simulink model "Sub2_2023"  (R2023b)
settings: Solver=FixedStepDiscrete  StartTime=0.0  StopTime=4.5  FixedStep=7.5e-05  RelTol=1e-3  EnableMultiTasking=on
undefined symbols (not defined in the file or in its folder): D1, D11, Delta
libraries: spsSeriesRLCBranchLib x41, spsLoadFlowBusLib x29, spsDistributedParametersLineLib x19, spsThreePhaseSeriesRLCLoadLib x15, spsThreePhaseTransformerTwoWindingsLib x13, spsThreePhaseParallelRLCLoadLib x11, spsThreePhaseVIMeasurementLib x11, spsSynchronousMachinepuStandardLib x7, spsExcitationSystemLib x7, spsHydraulicTurbineandGovernorLib x7, spsGenericPowerSystemStabilizerLib x7, spsMultiBandPowerSystemStabilizerLib x7
(part 2 of 5)

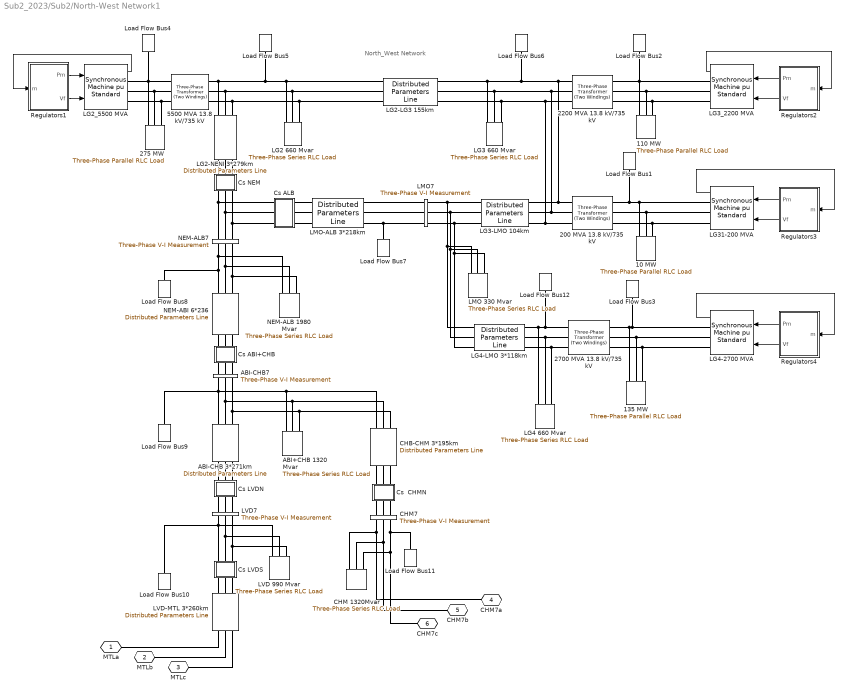
== system Sub2_2023/Sub2/North-West Network1 ==
  note: North_West Network
  10 MW : spsThreePhaseParallelRLCLoadLib/Three-Phase Parallel RLC Load  LConnTagsString=A|B|C  Configuration=Y (grounded)  NominalVoltage=(13800)*1  Vabc=[1e3 1e3 1e3]  Vabcp=[1e3 1e3 1e3]  NominalFrequency=60  UnbalancedPower=off  ActivePower=10000000  InductivePower=0  CapacitivePower=0  Pabc=[10e3 9e3 11e3]  QLabc=[100 90 110]  QCabc=[100 90 110]  Pabcp=[10e3 9e3 11e3]  QLabcp=[100 90 110]  QCabcp=[100 90 110]  Measurements=None  LoadType=constant PQ
  110 MW : spsThreePhaseParallelRLCLoadLib/Three-Phase Parallel RLC Load  LConnTagsString=A|B|C  Configuration=Y (grounded)  NominalVoltage=(13800)*1  Vabc=[1e3 1e3 1e3]  Vabcp=[1e3 1e3 1e3]  NominalFrequency=60  UnbalancedPower=off  ActivePower=110000000  InductivePower=0  CapacitivePower=0  Pabc=[10e3 9e3 11e3]  QLabc=[100 90 110]  QCabc=[100 90 110]  Pabcp=[10e3 9e3 11e3]  QLabcp=[100 90 110]  QCabcp=[100 90 110]  Measurements=None  LoadType=constant PQ
  135 MW : spsThreePhaseParallelRLCLoadLib/Three-Phase Parallel RLC Load  LConnTagsString=A|B|C  Configuration=Y (grounded)  NominalVoltage=(13800)*1  Vabc=[1e3 1e3 1e3]  Vabcp=[1e3 1e3 1e3]  NominalFrequency=60  UnbalancedPower=off  ActivePower=135000000  InductivePower=0  CapacitivePower=0  Pabc=[10e3 9e3 11e3]  QLabc=[100 90 110]  QCabc=[100 90 110]  Pabcp=[10e3 9e3 11e3]  QLabcp=[100 90 110]  QCabcp=[100 90 110]  Measurements=None  LoadType=constant PQ
  200 MVA 13.8 kV/735 kV : spsThreePhaseTransformerTwoWindingsLib/Three-Phase Transformer (Two Windings)  Winding1Connection=Delta (D1)  Winding2Connection=Yg  CoreType=Three single-phase transformers  SetSaturation=off  Hysteresis=off  DataFile='basic_model'  SetInitialFlux=off  Measurements=None  UNITS=pu  NominalPower=[ 200e6 60 ]  Winding1="[ 13.8e3 0.002  0.0]"  Winding2=[ 735e3 0.002 0.12]  Rm=500  Lm=500  L0=0.5  Saturation="[ 0,0  ;  0.005,1.2  ;  1.0,1.4 ]"  InitialFluxes=[ 0.8 , -0.8 , 0.7 ]  BreakLoop=off  DiscreteSolver=Trapezoidal iterative  DataType=off  TransfoNumber=0
  2200 MVA 13.8 kV/735 kV : spsThreePhaseTransformerTwoWindingsLib/Three-Phase Transformer (Two Windings)  Winding1Connection=Delta (D1)  Winding2Connection=Yg  CoreType=Three single-phase transformers  SetSaturation=off  Hysteresis=off  DataFile='basic_model'  SetInitialFlux=off  Measurements=None  UNITS=pu  NominalPower=[ 2200e6 60 ]  Winding1="[ 13.8e3 0.002  0.0]"  Winding2=[ 735e3 0.002 0.12]  Rm=500  Lm=500  L0=0.5  Saturation="[ 0,0  ;  0.005,1.2  ;  1.0,1.4 ]"  InitialFluxes=[ 0.8 , -0.8 , 0.7 ]  BreakLoop=off  DiscreteSolver=Trapezoidal iterative  DataType=off  TransfoNumber=0
  2700 MVA 13.8 kV/735 kV : spsThreePhaseTransformerTwoWindingsLib/Three-Phase Transformer (Two Windings)  Winding1Connection=Delta (D1)  Winding2Connection=Yg  CoreType=Three single-phase transformers  SetSaturation=off  Hysteresis=off  DataFile='basic_model'  SetInitialFlux=off  Measurements=None  UNITS=pu  NominalPower=[ 2700e6 60 ]  Winding1="[ 13.8e3 0.002  0.0]"  Winding2=[ 735e3 0.002 0.12]  Rm=500  Lm=500  L0=0.5  Saturation="[ 0,0  ;  0.005,1.2  ;  1.0,1.4 ]"  InitialFluxes=[ 0.8 , -0.8 , 0.7 ]  BreakLoop=off  DiscreteSolver=Trapezoidal iterative  DataType=off  TransfoNumber=0
  275 MW : spsThreePhaseParallelRLCLoadLib/Three-Phase Parallel RLC Load  LConnTagsString=A|B|C  Configuration=Y (grounded)  NominalVoltage=(13800)*1  Vabc=[1e3 1e3 1e3]  Vabcp=[1e3 1e3 1e3]  NominalFrequency=60  UnbalancedPower=off  ActivePower=275000000  InductivePower=0  CapacitivePower=0  Pabc=[10e3 9e3 11e3]  QLabc=[100 90 110]  QCabc=[100 90 110]  Pabcp=[10e3 9e3 11e3]  QLabcp=[100 90 110]  QCabcp=[100 90 110]  Measurements=None  LoadType=constant PQ
  5500 MVA 13.8 kV/735 kV : spsThreePhaseTransformerTwoWindingsLib/Three-Phase Transformer (Two Windings)  Winding1Connection=Delta (D1)  Winding2Connection=Yg  CoreType=Three single-phase transformers  SetSaturation=off  Hysteresis=off  DataFile='basic_model'  SetInitialFlux=off  Measurements=None  UNITS=pu  NominalPower=[ 5500e6 60 ]  Winding1="[ 13.8e3 0.002  0.0]"  Winding2=[ 735e3 0.002 0.12]  Rm=500  Lm=500  L0=0.5  Saturation="[ 0,0  ;  0.005,1.2  ;  1.0,1.4 ]"  InitialFluxes=[ 0.8 , -0.8 , 0.7 ]  BreakLoop=off  DiscreteSolver=Trapezoidal iterative  DataType=off  TransfoNumber=0
  ABI+CHB 1320 Mvar : spsThreePhaseSeriesRLCLoadLib/Three-Phase Series RLC Load  LConnTagsString=A|B|C  Configuration=Y (grounded)  NominalVoltage=735e3  Vabc=[1e3 1e3 1e3]  Vabcp=[1e3 1e3 1e3]  NominalFrequency=60  UnbalancedPower=off  ActivePower=4400000  InductivePower=1320e6  CapacitivePower=0  Pabc=[10e3 9e3 11e3]  QLabc=[100 90 110]  QCabc=[100 90 110]  Pabcp=[10e3 9e3 11e3]  QLabcp=[100 90 110]  QCabcp=[100 90 110]  Measurements=None  LoadType=constant Z
  ABI-CHB 3*271km : spsDistributedParametersLineLib/Distributed Parameters Line  Phases=3  Length=271  Frequency=60  Resistance="[0.01273  0.3864]/3"  Inductance="[0.9337e-3  4.1264e-3]/3"  Capacitance=[12.74e-9 7.751e-9]*3  x1=[-0.001575 2.6660325112539e-08 -34814.2579740654 -747194.944178159;-0.0015 2.67772386504407e-08 -13676.7298713687 -747880.497252828;-0.001425 2.68727468734707e-08 7471.73119992629 -747968.206100949;-0.00135 2.69467734338169e-08 28614.2194836213 -747458.00060941;-0.001275 2.69992591557795e-08 49733.8339980734 -746350.288628675;-0.0012 2.70301620830755e-08 70813.6920465805 -744645.955646752;-0.001125 2.70394575123777e-08 91836.9427131515 -742346.36408135;-0.00105 2.7027138013062e-08 112786.78033287 -739453.352190782;-0.000975 2.69932134331478e-08 133646.457926086 -735969.232604489;-0.0009 2.69377108914251e-08 154399.300585695 -731896.790474358;-0.000825 2.68606747557766e-08 175028.718806805 -727239.281248318;-0.00075 2.67621666077105e-08 195518.221748129 -722000.428067983;-0.000675 2.6642265193133e-08 215851.430414517 -716184.418792427;-0.0006 2.65010663594005e-08 236012.09075007 -709795.902650478;-0.000525 2.63386829787002e-08 255984.086631383 -702839.986524191;-0.00045 2.6155244857822e-08 275751.45275053 -695322.230866489;-0.000375 2.59508986343932e-08 295298.387377488 -687248.64525622;-0.0003 2.57258076596581e-08 314609.264991793 -678625.683594189;-0.000225 2.5480151867898e-08 333668.648773346 -669460.238944015;-0.00015 2.5214127632594e-08 352461.302942372 -659759.638021913;-7.5e-05 2.49279476094497e-08 370972.204938665 -649531.635339838]  x2=[-0.001575 6.10028275120772e-08 -284619.341076116 -691578.75825678;-0.0015 6.12059670998859e-08 -264954.25531131 -699348.683851085;-0.001425 6.13601795740777e-08 -245077.369168744 -706559.560807914;-0.00135 6.14653416595602e-08 -225004.571927074 -713205.624862556;-0.001275 6.15213692913713e-08 -204751.909473291 -719281.563253095;-0.0012 6.15282176818794e-08 -184335.571475885 -724782.518967347;-0.001125 6.1485881356586e-08 -163771.878443069 -729704.09462548;-0.00105 6.13943941585016e-08 -143077.268676419 -734042.355995217;-0.000975 6.12538292210926e-08 -122268.285130346 -737793.835136796;-0.0009 6.10642989098193e-08 -101361.562187906 -740955.533175191;-0.000825 6.08259547323125e-08 -80373.8123635378 -743524.922697366;-0.00075 6.05389872172611e-08 -59321.8129433265 -745499.949772649;-0.000675 6.02036257621058e-08 -38222.3925735024 -746879.035594615;-0.0006 5.98201384496626e-08 -17092.4178078773 -747661.077743159;-0.000525 5.93888318338216e-08 4051.22037502064 -747845.451065755;-0.00045 5.89100506944922e-08 25191.6200743366 -747432.008177186;-0.000375 5.83841777619916e-08 46311.8819780098 -746421.079577375;-0.0003 5.7811633411096e-08 67395.1228718253 -744813.473387174;-0.000225 5.71928753249992e-08 88424.4891355971 -742610.474702377;-0.00015 5.65283981294479e-08 109383.170215694 -739813.844566423;-7.5e-05 5.58187329973454e-08 130254.412063139 -736425.818562655]  x3=[-0.001575 1.20876651145068e-10 -354.964030660806 -109.750554356937;-0.0015 1.28668645904503e-10 -351.719210477191 -119.74113184108;-0.001425 1.36357784917099e-10 -348.193231338204 -129.635990096531;-0.00135 1.43937921602775e-10 -344.388911857622 -139.427219324996;-0.001275 1.51402996516247e-10 -340.309293150227 -149.106992567641;-0.0012 1.58747042190847e-10 -335.957636400794 -158.66757196184;-0.001125 1.65964187908831e-10 -331.337420257147 -168.101314926709;-0.00105 1.73048664394338e-10 -326.452338049379 -177.400680272461;-0.000975 1.79994808425261e-10 -321.306294837463 -186.558234228725;-0.0009 1.86797067360342e-10 -315.903404289605 -195.566656386983;-0.000825 1.93450003577867e-10 -310.247985393842 -204.418745552396;-0.00075 1.99948298822415e-10 -304.344559005508 -213.107425500326;-0.000675 2.06286758456196e-10 -298.197844233333 -221.625750632964;-0.0006 2.12460315611561e-10 -291.812754667058 -229.966911531533;-0.000525 2.18464035241378e-10 -285.194394449587 -238.124240399636;-0.00045 2.24293118064034e-10 -278.348054196814 -246.091216393387;-0.000375 2.2994290439991e-10 -271.279206768384 -253.861470834074;-0.0003 2.35408877896253e-10 -263.993502892774 -261.428792299187;-0.000225 2.40686669137482e-10 -256.496766650188 -268.787131587732;-0.00015 2.45772059138033e-10 -248.794990816874 -275.930606555866;-7.5e-05 2.50660982714947e-10 -240.894332074591 -282.853506818999]  x4=[-0.001575 1.8611765414938e-10 -5971.27343085196 -15054.8004559038;-0.0015 1.8231186212515e-10 -5543.27939856525 -15217.5948036283;-0.001425 1.78360332787803e-10 -5110.85415354235 -15368.2244389038;-0.00135 1.7426622492943e-10 -4674.3433699078 -15506.5689507045;-0.001275 1.70032811317211e-10 -4234.0959877032 -15632.5177485445;-0.0012 1.65663476077214e-10 -3790.46393394987 -15745.9701508819;-0.001125 1.61161711989177e-10 -3343.80184132378 -15846.8354656021;-0.00105 1.56531117694433e-10 -2894.46676466762 -15935.0330625157;-0.000975 1.51775394819211e-10 -2442.81789556661 -16010.4924378134;-0.0009 1.46898345015611e-10 -1989.21627521625 -16073.1532704251;-0.000825 1.41903866922626e-10 -1534.02450581152 -16122.9654702398;-0.00075 1.36795953049626e-10 -1077.6064606882 -16159.8892181473;-0.000675 1.31578686584805e-10 -620.326993448138 -16183.8949978684;-0.0006 1.2625623813115e-10 -162.551646300836 -16194.9636195501;-0.000525 1.20832862372518e-10 295.353642145395 -16193.0862351056;-0.00045 1.1531289467251e-10 753.022829409158 -16178.2643452873;-0.000375 1.09700747608848e-10 1210.09006174473 -16150.5097984871;-0.0003 1.04000907446025e-10 1666.18996659994 -16109.844781265;-0.000225 9.82179305490565e-11 2120.95794468941 -16056.3018006137;-0.00015 9.2356439741192e-11 2574.03046144964 -15989.9236579727;-7.5e-05 8.64211206084993e-11 3025.04533764297 -15910.7634150135]  x5=0.00153261764655846  V1=ones(3,3)  V2=ones(3,3)  I1=ones(3,3)  I2=ones(3,3)  nHarmo=1  Measurements=None  Decoupling=on  VsMag0=[610743.955114517 610743.501375054 610743.958218176]  VrMag0=[610622.360478052 610622.247686738 610622.214003776]  VsAngle0=[1.35232982185072 -118.647645266053 121.352379141739]  VrAngle0=[-18.3496130787589 -138.349622838574 101.65039120684]  IsMag0=[305.299965910612 305.301188711725 305.286778309069]  IrMag0=[13308.3117169369 13308.3164139137 13308.324626215]  IsAngle0=[-68.7963830005534 171.200626740077 51.201923119545]  IrAngle0=[-17.6151010152162 -137.615048514482 102.384907722651]
      settings: AttributesFormatString=\n  LibrarySourceBlock=sps_lib/Power Grid Elements/Distributed Parameters Line
  ABI-CHB7 : spsThreePhaseVIMeasurementLib/Three-Phase V-I Measurement  VoltageMeasurement=no  SetLabelV=on  LabelV=Vabc_ABI7  Vpu=on  VpuLL=off  CurrentMeasurement=no  SetLabelI=off  LabelI=A1  Ipu=off  Pbase=100e6  Vbase=500e3  OutputType=Magnitude  PhasorSimulation=off  PSBequivalent=0
  CHB-CHM 3*195km : spsDistributedParametersLineLib/Distributed Parameters Line  Phases=3  Length=195  Frequency=60  Resistance="[0.01273  0.3864]/3"  Inductance="[0.9337e-3  4.1264e-3]/3"  Capacitance=[12.74e-9 7.751e-9]*3  x1=[-0.001125 2.70394575123777e-08 0 0;-0.00105 2.7027138013062e-08 0 0;-0.000975 2.69932134331478e-08 0 0;-0.0009 2.69377108914251e-08 0 0;-0.000825 2.68606747557766e-08 0 0;-0.00075 2.67621666077105e-08 0 0;-0.000675 2.6642265193133e-08 215851.430414517 -716184.418792427;-0.0006 2.65010663594005e-08 236012.09075007 -709795.902650478;-0.000525 2.63386829787002e-08 255984.086631383 -702839.986524191;-0.00045 2.6155244857822e-08 275751.45275053 -695322.230866489;-0.000375 2.59508986343932e-08 295298.387377488 -687248.64525622;-0.0003 2.57258076596581e-08 314609.264991793 -678625.683594189;-0.000225 2.5480151867898e-08 333668.648773346 -669460.238944015;-0.00015 2.5214127632594e-08 352461.302942372 -659759.638021913;-7.5e-05 2.49279476094497e-08 370972.204938665 -649531.635339838]  x2=[-0.001125 1.81955879149765e-08 0 0;-0.00105 1.81407188523757e-08 0 0;-0.000975 1.80713483766866e-08 0 0;-0.0009 1.79875319416061e-08 0 0;-0.000825 1.788933654871e-08 0 0;-0.00075 1.77768406938928e-08 0 0;-0.000675 1.76501343046197e-08 127559.107191254 -726636.134488586;-0.0006 1.75093186680396e-08 148050.539525875 -722739.535823254;-0.000525 1.73545063500179e-08 168423.622524448 -718265.19023127;-0.00045 1.71858211051527e-08 188662.070256143 -713216.674436042;-0.000375 1.7003397777848e-08 208749.704415501 -707598.024143851;-0.0003 1.68073821945204e-08 228670.467255128 -701413.730817772;-0.000225 1.65979310470281e-08 248408.434422006 -694668.738087267;-0.00015 1.63752117674137e-08 267947.827687183 -687368.437796323;-7.5e-05 1.61394023940615e-08 287273.027558647 -679518.665693294]  x3=[-0.001125 1.00783620494122e-10 0 0;-0.00105 9.8868424952397e-11 0 0;-0.000975 9.68741955045023e-11 0 0;-0.0009 9.48025263069462e-11 0 0;-0.000825 9.26550734203876e-11 0 0;-0.00075 9.04335534858069e-11 0 0;-0.000675 8.81397423522494e-11 771.180648774861 -4323.83757003592;-0.0006 8.57754736572388e-11 893.110598565651 -4300.3071890933;-0.000525 8.33426373609954e-11 1014.326609409 -4273.33920838062;-0.00045 8.08431782356307e-11 1134.7317830805 -4242.95518568905;-0.000375 7.82790943105266e-11 1254.22986952659 -4209.17940954143;-0.0003 7.56524352751409e-11 1372.72534380533 -4172.03887977642;-0.000225 7.29653008405173e-11 1490.12348244765 -4131.56328596526;-0.00015 7.02198390608084e-11 1606.33043917774 -4087.78498367834;-7.5e-05 6.74182446161539e-11 1721.25331993244 -4040.73896862067]  x4=[-0.001125 7.25791212501294e-11 0 0;-0.00105 7.52447889614668e-11 0 0;-0.000975 7.78503071397922e-11 0 0;-0.0009 8.03935929737397e-11 0 0;-0.000825 8.28726133995272e-11 0 0;-0.00075 8.52853867261566e-11 0 0;-0.000675 8.76299842195474e-11 979.606952616618 -12037.6056406833;-0.0006 8.99045316443367e-11 1319.52443201694 -12005.1005057423;-0.000525 9.2107210762115e-11 1658.38710377571 -11962.9986771411;-0.00045 9.42362607848977e-11 1995.9240862579 -11911.3338104375;-0.000375 9.62899797826721e-11 2331.86555756419 -11850.1472057353;-0.0003 9.82667260438942e-11 2665.94297122251 -11779.4877746702;-0.000225 1.00164919387848e-10 2997.88927085992 -11699.4120013102;-0.00015 1.01983042427818e-10 3327.43910368346 -11609.9838970034;-7.5e-05 1.03719641784064e-10 3654.32903259903 -11511.274949208]  x5=0.0011028060556417  V1=ones(3,3)  V2=ones(3,3)  I1=ones(3,3)  I2=ones(3,3)  nHarmo=1  Measurements=None  Decoupling=on  VsMag0=[610743.955114517 610743.501375054 610743.958218176]  VrMag0=[602368.350238914 602368.356498701 602368.322152315]  VsAngle0=[1.35232982185072 -118.647645266053 121.352379141739]  VrAngle0=[-5.46332293595899 -125.46332636454 114.536674834106]  IsMag0=[3602.61669203481 3602.60152789078 3602.59275066962]  IrMag0=[9906.44607872251 9906.45414351813 9906.46948058419]  IsAngle0=[-5.30716137482798 -125.307461802343 114.692897272079]  IrAngle0=[-10.7676510977574 -130.767521740253 109.23237318601]
      settings: AttributesFormatString=\n  LibrarySourceBlock=sps_lib/Power Grid Elements/Distributed Parameters Line
  CHM 1320Mvar : spsThreePhaseSeriesRLCLoadLib/Three-Phase Series RLC Load  LConnTagsString=A|B|C  Configuration=Y (grounded)  NominalVoltage=735e3  Vabc=[1e3 1e3 1e3]  Vabcp=[1e3 1e3 1e3]  NominalFrequency=60  UnbalancedPower=off  ActivePower=4400000  InductivePower=1320e6  CapacitivePower=0  Pabc=[10e3 9e3 11e3]  QLabc=[100 90 110]  QCabc=[100 90 110]  Pabcp=[10e3 9e3 11e3]  QLabcp=[100 90 110]  QCabcp=[100 90 110]  Measurements=None  LoadType=constant Z
  CHM7 : spsThreePhaseVIMeasurementLib/Three-Phase V-I Measurement  VoltageMeasurement=no  SetLabelV=on  LabelV=Vabc_CHM7  Vpu=on  VpuLL=off  CurrentMeasurement=no  SetLabelI=off  LabelI=A1  Ipu=off  Pbase=100e6  Vbase=735e3  OutputType=Magnitude  PhasorSimulation=off  PSBequivalent=0
  "Cs  CHMN " : Subsystem  mask{Xc=25/3}
      mask prompts: Xc "Condensator Reactance at  60Hz  (ohm):"
      mask help: Series Compensation
      mask init:
      | Cs=1/Xc/(2*pi*60);
      mask Display: disp('Cs')
  "Cs ABI+CHB " : Subsystem  mask{Xc=25/6}
      mask prompts: Xc "Condensator Reactance at  60Hz  (ohm):"
      mask help: Series Compensation
      mask init:
      | Cs=1/Xc/(2*pi*60);
      mask Display: disp('Cs')
  Cs ALB : Subsystem  mask{Xc=16/3}
      mask prompts: Xc "Reactance @ 60Hz du condensateur (ohm):"
      mask init:
      | Cs=1/Xc/(2*pi*60);
      mask Display: disp('Cs')
  "Cs LVDN " : Subsystem  mask{Xc=34/3}
      mask prompts: Xc "Condensator Reactance at  60Hz  (ohm):"
      mask help: Series Compensation
      mask init:
      | Cs=1/Xc/(2*pi*60);
      mask Display: disp('Cs')
  "Cs LVDS " : Subsystem  mask{Xc=34/3}
      mask prompts: Xc "Condensator Reactance at  60Hz  (ohm):"
      mask help: Series Compensation
      mask init:
      | Cs=1/Xc/(2*pi*60);
      mask Display: disp('Cs')
  "Cs NEM " : Subsystem  mask{Xc=16/3}
      mask prompts: Xc "Condensator Reactance at  60Hz  (ohm):"
      mask help: Series Compensation
      mask init:
      | Cs=1/Xc/(2*pi*60);
      mask Display: disp('Cs')
  LG2 660 Mvar : spsThreePhaseSeriesRLCLoadLib/Three-Phase Series RLC Load  LConnTagsString=A|B|C  Configuration=Y (grounded)  NominalVoltage=735e3  Vabc=[1e3 1e3 1e3]  Vabcp=[1e3 1e3 1e3]  NominalFrequency=60  UnbalancedPower=off  ActivePower=2200000  InductivePower=660e6  CapacitivePower=0  Pabc=[10e3 9e3 11e3]  QLabc=[100 90 110]  QCabc=[100 90 110]  Pabcp=[10e3 9e3 11e3]  QLabcp=[100 90 110]  QCabcp=[100 90 110]  Measurements=None  LoadType=constant Z
  LG2-LG3 155km : spsDistributedParametersLineLib/Distributed Parameters Line  Phases=3  Length=155  Frequency=60  Resistance="[0.01273  0.3864]"  Inductance="[0.9337e-3  4.1264e-3]"  Capacitance=[12.74e-9 7.751e-9]  x1=[-0.0009 4.79474772159392e-10 425726.576739838 -584301.004479771;-0.000825 5.22458298158404e-10 442074.911234261 -572031.872778104;-0.00075 5.65024178987748e-10 458069.857808617 -559305.46754972;-0.000675 6.0713838813357e-10 473698.630347344 -546131.962088236;-0.0006 6.48767260141446e-10 488948.735448804 -532521.887092359;-0.000525 6.89877517528037e-10 503807.982412312 -518486.122247798;-0.00045 7.30436297382596e-10 518264.492983201 -504035.887530215;-0.000375 7.70411177637078e-10 532306.710848112 -489182.734236149;-0.0003 8.09770202983843e-10 545923.410872936 -473938.535749081;-0.000225 8.48481910420242e-10 559103.708076017 -458315.478048038;-0.00015 8.8651535439966e-10 571837.066329435 -442326.049966306;-7.5e-05 9.2384013156891e-10 584113.30678143 -425983.033208046]  x2=[-0.0009 -3.11578283864764e-10 428602.512418884 -576982.581433748;-0.000825 -3.58188817976031e-10 444742.801992352 -564635.073574132;-0.00075 -4.04513021426679e-10 460527.5709747 -551836.205075907;-0.000675 -4.50513863357257e-10 475944.201263119 -538596.207158722;-0.0006 -4.96154571398559e-10 490980.369039239 -524925.663674332;-0.000525 -5.41398661066906e-10 505624.0546206 -510835.502646033;-0.00045 -5.86209964929272e-10 519863.552069006 -496336.987532963;-0.000375 -6.30552661514988e-10 533687.478548066 -481441.708226271;-0.0003 -6.74391303950867e-10 547084.783422467 -466161.571784328;-0.000225 -7.17690848296901e-10 560044.757091678 -450508.792914411;-0.00015 -7.60416681559845e-10 572557.039551043 -434495.884208455;-7.5e-05 -8.02534649362315e-10 584611.628673407 -418135.646140672]  x3=[-0.0009 1.2171764561214e-11 1482.81916403306 -2352.94053779613;-0.000825 1.20724465253453e-11 1548.74539245901 -2310.07973089156;-0.00075 1.19634779604388e-11 1613.43357751482 -2265.37228159552;-0.000675 1.1844945974298e-11 1676.83200845514 -2218.85392835893;-0.0006 1.17169453195792e-11 1738.89000554428 -2170.56185724162;-0.000525 1.15795783180472e-11 1799.55796056891 -2120.53467218633;-0.00045 1.14329547787812e-11 1858.78737649401 -2068.81236415937;-0.000375 1.12771919103952e-11 1916.53090623075 -2015.43627918239;-0.0003 1.11124142273428e-11 1972.74239048495 -1960.44908528104;-0.000225 1.09387534503827e-11 2027.37689465617 -1903.8947383768;-0.00015 1.07563484012829e-11 2080.3907447577 -1845.81844714926;-7.5e-05 1.05653448918487e-11 2131.74156232893 -1786.26663689704]  x4=[-0.0009 -1.22867634504129e-11 1223.55408119269 -2231.14873574853;-0.000825 -1.21689195399199e-11 1286.14070278682 -2195.66620561517;-0.00075 -1.20413479813375e-11 1347.69920318175 -2158.42849351186;-0.000675 -1.19041507534175e-11 1408.18037345415 -2119.46536669589;-0.0006 -1.17574375295249e-11 1467.53586588189 -2078.8079716947;-0.000525 -1.1601325589966e-11 1525.7182325925 -2036.48880940776;-0.00045 -1.14359397282367e-11 1582.68096349224 -1992.54170912591;-0.000375 -1.12614121512644e-11 1638.3785234456 -1947.00180148869;-0.0003 -1.10778823737237e-11 1692.76638867535 -1899.90549040149;-0.000225 -1.08854971065108e-11 1745.80108235419 -1851.29042393479;-0.00015 -1.06844101394647e-11 1797.44020935944 -1801.19546422889;-7.5e-05 -1.047478221843e-11 1847.64249016309 -1749.6606564281]  x5=0.000876589428843401  V1=ones(3,3)  V2=ones(3,3)  I1=ones(3,3)  I2=ones(3,3)  nHarmo=1  Measurements=None  Decoupling=on  VsMag0=[590283.05661736 590282.243891932 590283.870916954]  VrMag0=[586861.315379263 586860.569064607 586862.120536263]  VsAngle0=[25.5173905041417 -94.4824726828106 145.517527228784]  VrAngle0=[26.0462334057209 -93.9536337576133 146.046362925435]  IsMag0=[2279.13376434119 2279.13000762796 2279.13554694091]  IrMag0=[2085.26033535307 2085.25824212163 2085.2645601678]  IsAngle0=[21.6590596698336 -98.340834058637 141.659194593849]  IrAngle0=[18.1802070278252 -101.819625724327 138.180340460882]
      settings: AttributesFormatString=\n  LibrarySourceBlock=sps_lib/Power Grid Elements/Distributed Parameters Line
  LG2-NENI 3*279km : spsDistributedParametersLineLib/Distributed Parameters Line  Phases=3  Length=279  Frequency=60  Resistance="[0.01273  0.3864]/3"  Inductance="[0.9337e-3  4.1264e-3]/3"  Capacitance=[12.74e-9 7.751e-9]*3  x1=[-0.00165 3.43578378924508e-11 245808.020606819 -679875.080306934;-0.001575 7.95866779331643e-11 264930.184927482 -672654.157661494;-0.0015 1.24751897601255e-10 283840.568111882 -664895.525574374;-0.001425 1.69817392511172e-10 302524.05348904 -656605.386177352;-0.00135 2.14747137995808e-10 320965.705766612 -647790.366481019;-0.001275 2.59505217904072e-10 339150.782969934 -638457.513077247;-0.0012 3.04055853311706e-10 357064.748226531 -628614.286506247;-0.001125 3.48363431122413e-10 374693.281386669 -618268.555292737;-0.00105 3.92392532536421e-10 392022.290470667 -607428.589655951;-0.000975 4.36107961363726e-10 409037.922933804 -596103.054898563;-0.0009 4.79474772159392e-10 425726.576739838 -584301.004479771;-0.000825 5.22458298158404e-10 442074.911234261 -572031.872778104;-0.00075 5.65024178987748e-10 458069.857808617 -559305.46754972;-0.000675 6.0713838813357e-10 473698.630347344 -546131.962088236;-0.0006 6.48767260141446e-10 488948.735448804 -532521.887092359;-0.000525 6.89877517528037e-10 503807.982412312 -518486.122247798;-0.00045 7.30436297382596e-10 518264.492983201 -504035.887530215;-0.000375 7.70411177637078e-10 532306.710848112 -489182.734236149;-0.0003 8.09770202983843e-10 545923.410872936 -473938.535749081;-0.000225 8.48481910420242e-10 559103.708076017 -458315.478048038;-0.00015 8.8651535439966e-10 571837.066329435 -442326.049966306;-7.5e-05 9.2384013156891e-10 584113.30678143 -425983.033208046]  x2=[-0.00165 1.53679119664061e-08 25617.0786733969 -737924.872189153;-0.001575 1.54505402786779e-08 46468.3767747066 -736905.697758638;-0.0015 1.55208176654522e-08 67282.5287666127 -735297.452188371;-0.001425 1.55786879480612e-08 88042.89613448 -733101.421085252;-0.00135 1.56241048658864e-08 108732.883358279 -730319.359922946;-0.001275 1.56570321133387e-08 129335.95117879 -726953.492638578;-0.0012 1.56774433688802e-08 149835.629818835 -723006.509854957;-0.001125 1.56853223160655e-08 170215.532148965 -718481.566729728;-0.00105 1.56806626565849e-08 190459.36678708 -713382.280433191;-0.000975 1.56634681152987e-08 210550.951121512 -707712.727256792;-0.0009 1.56337524372603e-08 230474.224247155 -701477.439354591;-0.000825 1.5591539376728e-08 250213.259804308 -694681.401120335;-0.00075 1.55368626781764e-08 269752.278709965 -687330.045203005;-0.000675 1.54697660493219e-08 289075.661771369 -679429.248164042;-0.0006 1.5390303126183e-08 308167.96217176 -670985.325779713;-0.000525 1.52985374302045e-08 327013.917818318 -662005.027992375;-0.00045 1.51945423174797e-08 345598.463542453 -652495.533514677;-0.000375 1.50784009201107e-08 363906.743142666 -642464.444091004;-0.0003 1.49502060797534e-08 381924.121260371 -631919.77842076;-0.000225 1.48100602734018e-08 399636.195079175 -620869.965748343;-0.00015 1.46580755314691e-08 417028.805838272 -609323.839124936;-7.5e-05 1.44943733482327e-08 434088.050150736 -597290.6283475]  x3=[-0.00165 9.42442462266143e-12 -714.300687612593 -1196.52974167988;-0.001575 1.23583898062467e-11 -680.188293409888 -1216.24398928775;-0.0015 1.52824758821106e-11 -645.53216709266 -1234.98599005975;-0.001425 1.81943453805841e-11 -610.360012238032 -1252.74076192721;-0.00135 2.10916705977432e-11 -574.699944928442 -1269.49411199716;-0.001275 2.39721354561397e-11 -538.58047127608 -1285.23264789789;-0.0012 2.68334373562387e-11 -502.030464635538 -1299.94378848462;-0.001125 2.96732890170804e-11 -465.07914252289 -1313.61577389663;-0.00105 3.24894203046984e-11 -427.756043259659 -1326.23767495799;-0.000975 3.52795800468296e-11 -390.091002360332 -1337.7994019141;-0.0009 3.80415378324671e-11 -352.114128682312 -1348.29171249734;-0.000825 4.07730857948163e-11 -313.855780357349 -1357.70621931517;-0.00075 4.34720403762303e-11 -275.346540523724 -1366.03539655487;-0.000675 4.61362440737121e-11 -236.617192878547 -1373.27258599962;-0.0006 4.87635671635895e-11 -197.698697069747 -1379.41200235089;-0.000525 5.1351909403984e-11 -158.622163947402 -1384.44873785319;-0.00045 5.38992017137114e-11 -119.418830694197 -1388.37876621722;-0.000375 5.64034078262744e-11 -80.1200358549047 -1391.19894583846;-0.0003 5.88625259176222e-11 -40.7571942848277 -1392.90702230844;-0.000225 6.12745902063782e-11 -1.36177203724539 -1393.50163021699;-0.00015 6.36376725252559e-11 38.0347387900677 -1392.98229424362;-7.5e-05 6.5949883862406e-11 77.4008452291431 -1391.34942953759]  x4=[-0.00165 3.9116821997204e-11 829.758142042443 -14907.5065102238;-0.001575 3.69850672272189e-11 1250.86903709572 -14878.0908857497;-0.0015 3.48237471603829e-11 1670.98000657968 -14836.7819430639;-0.001425 3.2634589522888e-11 2089.75522021323 -14783.6127039033;-0.00135 3.04193442938545e-11 2506.85991549807 -14718.625670944;-0.001275 2.81797823064241e-11 2921.9606653227 -14641.8727938259;-0.0012 2.59176938321831e-11 3334.72564449897 -14553.4154276246;-0.001125 2.36348871500466e-11 3744.82489501805 -14453.3242838051;-0.00105 2.13331871007483e-11 4151.93058981378 -14341.6793736965;-0.000975 1.90144336280903e-11 4555.71729482269 -14218.5699445316;-0.0009 1.66804803081206e-11 4955.86222913093 -14084.0944081044;-0.000825 1.43331928674126e-11 5352.04552300044 -13938.3602621013;-0.00075 1.19744476916315e-11 5743.9504735679 -13781.4840041687;-0.000675 9.60613032558093e-12 6131.26379801219 -13613.5910387869;-0.0006 7.23013396592682e-12 6513.67588398782 -13434.8155770237;-0.000525 4.84835794780511e-12 6890.88103712437 -13245.3005292477;-0.00045 2.46270622652228e-12 7262.57772539387 -13045.1973908886;-0.000375 7.50858555626392e-14 7628.46882015085 -12834.6661213334;-0.0003 -2.31259453788109e-12 7988.26183365249 -12613.8750160578;-0.000225 -4.69842627863511e-12 8341.66915286881 -12383.0005720932;-0.00015 -7.08050216931033e-12 8688.40826939614 -12142.2273469374;-7.5e-05 -9.45691801488672e-12 9028.20200529003 -11891.7478110228]  x5=0.00157786097191812  V1=ones(3,3)  V2=ones(3,3)  I1=ones(3,3)  I2=ones(3,3)  nHarmo=1  Measurements=None  Decoupling=on  VsMag0=[590283.05661736 590282.243891932 590283.870916954]  VrMag0=[602875.980203761 602875.44101502 602876.102194797]  VsAngle0=[25.5173905041417 -94.4824726828106 145.517527228784]  VrAngle0=[7.62822080531618 -112.371736222193 127.628286669376]  IsMag0=[1145.30812027456 1145.28643710015 1145.27794996468]  IrMag0=[12270.9673380093 12270.9820903555 12270.998354888]  IsAngle0=[-25.1951184882616 -145.19623504081 94.8052626724784]  IrAngle0=[8.82574494857365 -111.17412759158 128.825749025237]
      settings: AttributesFormatString=\n  LibrarySourceBlock=sps_lib/Power Grid Elements/Distributed Parameters Line
  LG2_5500 MVA : spsSynchronousMachinepuStandardLib/Synchronous Machine pu Standard  PresetModel=No  MechanicalLoad=Mechanical power Pm  ShowDetailedParameters=on  RotorType=Salient-pole  Units=per unit standard parameters  MeasurementBus=off  NominalParameters="[5500E6  13800   60 ]"  Reactances1=[ 31 32 33 34 35 36 37 ]  Reactances2=[ 1.305, 0.296, 0.252, 0.474, 0.243, 0.18 ]  dAxisTimeConstants=Short-circuit  qAxisTimeConstants=Open-circuit  TimeConstants1=[]  TimeConstants2=[]  TimeConstants3=[]  TimeConstants4=[]  TimeConstants5=[ 1.01, 0.053, 0.1 ]  TimeConstants6=[]  TimeConstants7=[]  TimeConstants8=[]  StatorResistance=2.8544e-3  Mechanical="[ 4.1  0  32]"  PolePairs=32  InitialConditions=[0 -65.2434 0.985682 0.985682 0.985682 -1.22427 -121.224 118.776 1.47412]  SetSaturation=off  Saturation=[0.6404,0.7127,0.8441,0.9214,0.9956,1.082,1.19,1.316,1.457;0.7,0.7698,0.8872,0.9466,0.9969,1.046,1.1,1.151,1.201]  LoadFlowParameters=[2 4000000000 0 0 0]  TsPowergui=0  TsBlock=-1  IterativeModel=Trapezoidal non iterative  IterativeDiscreteModel=Trapezoidal non iterative  BusType=swing  Pref=0  Qref=0  Qmin=-Inf  Qmax=Inf  PLF=0  QLF=0
  LG3 660 Mvar : spsThreePhaseSeriesRLCLoadLib/Three-Phase Series RLC Load  LConnTagsString=A|B|C  Configuration=Y (grounded)  NominalVoltage=735e3  Vabc=[1e3 1e3 1e3]  Vabcp=[1e3 1e3 1e3]  NominalFrequency=60  UnbalancedPower=off  ActivePower=2200000  InductivePower=660e6  CapacitivePower=0  Pabc=[10e3 9e3 11e3]  QLabc=[100 90 110]  QCabc=[100 90 110]  Pabcp=[10e3 9e3 11e3]  QLabcp=[100 90 110]  QCabcp=[100 90 110]  Measurements=None  LoadType=constant Z
  LG3-LMO 104km : spsDistributedParametersLineLib/Distributed Parameters Line  Phases=3  Length=104  Frequency=60  Resistance="[0.01273  0.3864]"  Inductance="[0.9337e-3  4.1264e-3]"  Capacitance=[12.74e-9 7.751e-9]  x1=[-0.0006 -4.96154571398559e-10 0 0;-0.000525 -5.41398661066906e-10 0 0;-0.00045 -5.86209964929272e-10 0 0;-0.000375 -6.30552661514988e-10 533687.478548066 -481441.708226271;-0.0003 -6.74391303950867e-10 547084.783422467 -466161.571784328;-0.000225 -7.17690848296901e-10 560044.757091678 -450508.792914411;-0.00015 -7.60416681559845e-10 572557.039551043 -434495.884208455;-7.5e-05 -8.02534649362315e-10 584611.628673407 -418135.646140672]  x2=[-0.0006 4.32429146837349e-09 0 0;-0.000525 4.25360370502354e-09 0 0;-0.00045 4.17951567595412e-09 0 0;-0.000375 4.10208660600207e-09 480200.396912808 -552194.743514957;-0.0003 4.02137839078122e-09 495619.314773644 -538398.460516582;-0.000225 3.93745554720392e-09 510642.04213748 -524171.790026643;-0.00015 3.85038516190729e-09 525256.570065916 -509526.104627854;-7.5e-05 3.76023683762509e-09 539451.215928937 -494473.111857036]  x3=[-0.0006 1.46588171322479e-11 0 0;-0.000525 1.52954631842922e-11 0 0;-0.00045 1.59198822770954e-11 0 0;-0.000375 1.65315752595887e-11 -139.986222681468 -514.51577923704;-0.0003 1.71300531537611e-11 -125.384058316405 -518.267255560566;-0.000225 1.77148375455409e-11 -110.681663853565 -521.604436969753;-0.00015 1.82854609672329e-11 -95.8907921621266 -524.524655772841;-7.5e-05 1.88414672712047e-11 -81.0232668386119 -527.025577591601]  x4=[-0.0006 -6.59927454528263e-12 0 0;-0.000525 -7.40317436164863e-12 0 0;-0.00045 -8.20115619370228e-12 0 0;-0.000375 -8.99258214697659e-12 3613.50960647482 -3542.58660366534;-0.0003 -9.77681956767373e-12 3712.21557844748 -3439.01470479912;-0.000225 -1.05532415483988e-11 3807.95406208553 -3332.69371019658;-0.00015 -1.13212274293001e-11 3900.64852551 -3223.70861123403;-7.5e-05 -1.20801632942151e-11 3990.2248701851 -3112.14652893206]  x5=0.000588163229675572  V1=ones(3,3)  V2=ones(3,3)  I1=ones(3,3)  I2=ones(3,3)  nHarmo=1  Measurements=None  Decoupling=on  VsMag0=[586861.315379263 586860.569064607 586862.120536263]  VrMag0=[597501.495499285 597500.918482545 597501.873521954]  VsAngle0=[26.0462334057209 -93.9536337576133 146.046362925435]  VrAngle0=[19.1109154470688 -100.889010750014 139.11100026692]  IsMag0=[436.451079902145 436.445924432093 436.434679859544]  IrMag0=[4141.87607401762 4141.88820061795 4141.89211373257]  IsAngle0=[-37.1184575597095 -157.120552819953 82.8810809575937]  IrAngle0=[23.6678939917951 -96.3319466522286 143.66782839401]
      settings: AttributesFormatString=\n  LibrarySourceBlock=sps_lib/Power Grid Elements/Distributed Parameters Line
  LG31-200 MVA : spsSynchronousMachinepuStandardLib/Synchronous Machine pu Standard  PresetModel=No  MechanicalLoad=Mechanical power Pm  ShowDetailedParameters=on  RotorType=Salient-pole  Units=per unit standard parameters  MeasurementBus=off  NominalParameters="[200E6  13800   60 ]"  Reactances1=[ 31 32 33 34 35 36 37 ]  Reactances2=[ 1.305, 0.296, 0.252, 0.474, 0.243, 0.18 ]  dAxisTimeConstants=Short-circuit  qAxisTimeConstants=Open-circuit  TimeConstants1=[]  TimeConstants2=[]  TimeConstants3=[]  TimeConstants4=[]  TimeConstants5=[ 1.01, 0.053, 0.1 ]  TimeConstants6=[]  TimeConstants7=[]  TimeConstants8=[]  StatorResistance=2.8544e-3  Mechanical="[ 3.2  0  32]"  PolePairs=32  InitialConditions=[0 -67.6291 0.902477 0.902477 0.902477 -4.2812 -124.281 115.719 1.45511]  SetSaturation=off  Saturation=[0.6404,0.7127,0.8441,0.9214,0.9956,1.082,1.19,1.316,1.457;0.7,0.7698,0.8872,0.9466,0.9969,1.046,1.1,1.151,1.201]  LoadFlowParameters=[1 180000000 0 0 0]  TsPowergui=0  TsBlock=-1  IterativeModel=Trapezoidal non iterative  IterativeDiscreteModel=Trapezoidal non iterative  BusType=PV  Pref=180000000  Qref=0  Qmin=-Inf  Qmax=Inf  PLF=0  QLF=0
  LG3_2200 MVA : spsSynchronousMachinepuStandardLib/Synchronous Machine pu Standard  PresetModel=No  MechanicalLoad=Mechanical power Pm  ShowDetailedParameters=on  RotorType=Salient-pole  Units=per unit standard parameters  MeasurementBus=off  NominalParameters="[2200E6  13800   60 ]"  Reactances1=[ 31 32 33 34 35 36 37 ]  Reactances2=[ 1.305, 0.296, 0.252, 0.474, 0.243, 0.18 ]  dAxisTimeConstants=Short-circuit  qAxisTimeConstants=Open-circuit  TimeConstants1=[]  TimeConstants2=[]  TimeConstants3=[]  TimeConstants4=[]  TimeConstants5=[ 1.01, 0.053, 0.1 ]  TimeConstants6=[]  TimeConstants7=[]  TimeConstants8=[]  StatorResistance=2.8544e-3  Mechanical="[ 3.2  0  32]"  PolePairs=32  InitialConditions=[0 -70.0065 0.820496 0.820496 0.820496 -4.90643 -124.906 115.094 1.38903]  SetSaturation=off  Saturation=[0.6404,0.7127,0.8441,0.9214,0.9956,1.082,1.19,1.316,1.457;0.7,0.7698,0.8872,0.9466,0.9969,1.046,1.1,1.151,1.201]  LoadFlowParameters=[1 1800000000 0 0 0]  TsPowergui=0  TsBlock=-1  IterativeModel=Trapezoidal non iterative  IterativeDiscreteModel=Trapezoidal non iterative  BusType=PV  Pref=1800000000  Qref=0  Qmin=-Inf  Qmax=Inf  PLF=0  QLF=0
  LG4 660 Mvar : spsThreePhaseSeriesRLCLoadLib/Three-Phase Series RLC Load  LConnTagsString=A|B|C  Configuration=Y (grounded)  NominalVoltage=735e3  Vabc=[1e3 1e3 1e3]  Vabcp=[1e3 1e3 1e3]  NominalFrequency=60  UnbalancedPower=off  ActivePower=2200000  InductivePower=660e6  CapacitivePower=0  Pabc=[10e3 9e3 11e3]  QLabc=[100 90 110]  QCabc=[100 90 110]  Pabcp=[10e3 9e3 11e3]  QLabcp=[100 90 110]  QCabcp=[100 90 110]  Measurements=None  LoadType=constant Z
  LG4-2700 MVA : spsSynchronousMachinepuStandardLib/Synchronous Machine pu Standard  PresetModel=No  MechanicalLoad=Mechanical power Pm  ShowDetailedParameters=on  RotorType=Salient-pole  Units=per unit standard parameters  MeasurementBus=off  NominalParameters="[2700E6  13800   60 ]"  Reactances1=[ 31 32 33 34 35 36 37 ]  Reactances2=[ 1.305, 0.296, 0.252, 0.474, 0.243, 0.18 ]  dAxisTimeConstants=Short-circuit  qAxisTimeConstants=Open-circuit  TimeConstants1=[]  TimeConstants2=[]  TimeConstants3=[]  TimeConstants4=[]  TimeConstants5=[ 1.01, 0.053, 0.1 ]  TimeConstants6=[]  TimeConstants7=[]  TimeConstants8=[]  StatorResistance=2.8544e-3  Mechanical="[ 3.7  0  32]"  PolePairs=32  InitialConditions=[0 -69.506 0.926038 0.926038 0.926038 -2.40174 -122.402 117.598 1.38766]  SetSaturation=off  Saturation=[0.6404,0.7127,0.8441,0.9214,0.9956,1.082,1.19,1.316,1.457;0.7,0.7698,0.8872,0.9466,0.9969,1.046,1.1,1.151,1.201]  LoadFlowParameters=[1 2500000000 0 0 0]  TsPowergui=0  TsBlock=-1  IterativeModel=Trapezoidal non iterative  IterativeDiscreteModel=Trapezoidal non iterative  BusType=PV  Pref=2500000000  Qref=0  Qmin=-Inf  Qmax=Inf  PLF=0  QLF=0
  LG4-LMO 3*118km : spsDistributedParametersLineLib/Distributed Parameters Line  Phases=3  Length=118  Frequency=60  Resistance="[0.01273  0.3864]/3"  Inductance="[0.9337e-3  4.1264e-3]/3"  Capacitance=[12.74e-9 7.751e-9]*3  x1=[-0.000675 -6.13819447065466e-10 446066.324942447 -570785.422694684;-0.0006 -6.77598921029316e-10 462024.453036369 -557946.7066079;-0.000525 -7.40836732783308e-10 477613.245851745 -544661.976460724;-0.00045 -8.03482330988294e-10 492820.241946115 -530941.851863174;-0.000375 -8.6548563771158e-10 507633.285079476 -516797.300472926;-0.0003 -9.26797088458454e-10 522040.533931794 -502239.629227945;-0.000225 -9.87367671793285e-10 536030.471568775 -487280.475307883;-0.00015 -1.04714896851852e-09 549591.914648326 -471931.7968315;-7.5e-05 -1.10609319038023e-09 562714.022360344 -456205.86329753]  x2=[-0.000675 4.39152245928749e-09 414813.87544859 -602860.773675277;-0.0006 4.32429146837349e-09 431691.280998714 -590892.75502538;-0.000525 4.25360370502354e-09 448223.599143905 -578452.385748079;-0.00045 4.17951567595412e-09 464397.614201993 -565549.610484229;-0.000375 4.10208660600207e-09 480200.396912808 -552194.743514957;-0.0003 4.02137839078122e-09 495619.314773644 -538398.460516582;-0.000225 3.93745554720392e-09 510642.04213748 -524171.790026643;-0.00015 3.85038516190729e-09 525256.570065916 -509526.104627854;-7.5e-05 3.76023683762509e-09 539451.215928937 -494473.111857036]  x3=[-0.000675 1.39167840064082e-11 2040.14143601601 -4504.23210447826;-0.0006 1.57645670394048e-11 2166.66257243637 -4444.75566915328;-0.000525 1.7599748118716e-11 2291.45171194738 -4381.72616415343;-0.00045 1.94208602286664e-11 2414.40910002024 -4315.1939743006;-0.000375 2.1226447600099e-11 2535.43644640025 -4245.21228440941;-0.0003 2.30150668740957e-11 2654.43700367848 -4171.83703677198;-0.000225 2.47852882557756e-11 2771.31564463022 -4095.1268864386;-0.00015 2.65356966572514e-11 2885.97893825819 -4015.14315432975;-7.5e-05 2.82648928288292e-11 2998.33522447988 -3931.94977821707]  x4=[-0.000675 8.56540692443732e-14 6463.18076750046 -9178.78456746962;-0.0006 -2.39863931994355e-12 6720.08725258113 -8992.39755657967;-0.000525 -4.88101527355954e-12 6971.62180273286 -8798.82216067128;-0.00045 -7.35948941824787e-12 7217.58334508489 -8598.21312095415;-0.000375 -9.83208049969922e-12 7457.77526174358 -8390.73080122519;-0.0003 -1.2296811966435e-11 7692.00554696582 -8176.54105967623;-0.000225 -1.47517135498323e-11 7920.08696064545 -7955.81511630943;-0.00015 -1.71948228391267e-11 8141.83717799013 -7728.72941606671;-7.5e-05 -1.96241868501331e-11 8357.07893526902 -7495.46548778231]  x5=0.000667339049054976  V1=ones(3,3)  V2=ones(3,3)  I1=ones(3,3)  I2=ones(3,3)  nHarmo=1  Measurements=None  Decoupling=on  VsMag0=[591479.207020492 591478.775968516 591479.558478893]  VrMag0=[597501.495499285 597500.918482545 597501.873521954]  VsAngle0=[22.5874691411624 -97.4124674391999 142.587537012198]  VrAngle0=[19.1109154470688 -100.889010750014 139.11100026692]  IsMag0=[4048.55267184838 4048.55521766257 4048.56794770048]  IrMag0=[9191.4611750621 9191.44543051444 9191.45421674983]  IsAngle0=[8.94759792223368 -111.052173248438 128.947681135212]  IrAngle0=[19.7310305258183 -100.268962895621 139.731118811241]
      settings: AttributesFormatString=\n  LibrarySourceBlock=sps_lib/Power Grid Elements/Distributed Parameters Line
  LMO 330 Mvar : spsThreePhaseSeriesRLCLoadLib/Three-Phase Series RLC Load  LConnTagsString=A|B|C  Configuration=Y (grounded)  NominalVoltage=735e3  Vabc=[1e3 1e3 1e3]  Vabcp=[1e3 1e3 1e3]  NominalFrequency=60  UnbalancedPower=off  ActivePower=1100000  InductivePower=330e6  CapacitivePower=0  Pabc=[10e3 9e3 11e3]  QLabc=[100 90 110]  QCabc=[100 90 110]  Pabcp=[10e3 9e3 11e3]  QLabcp=[100 90 110]  QCabcp=[100 90 110]  Measurements=None  LoadType=constant Z
  LMO-ALB 3*218km : spsDistributedParametersLineLib/Distributed Parameters Line  Phases=3  Length=218  Frequency=60  Resistance="[0.01273  0.3864]/3"  Inductance="[0.9337e-3  4.1264e-3]/3"  Capacitance=[12.74e-9 7.751e-9]*3  x1=[-0.001275 4.79907646041783e-09 0 0;-0.0012 4.76119384583493e-09 0 0;-0.001125 4.71950520574038e-09 0 0;-0.00105 4.67404386539522e-09 0 0;-0.000975 4.62484616589932e-09 0 0;-0.0009 4.57195143514093e-09 0 0;-0.000825 4.51540195635848e-09 380078.033365262 -625341.876126506;-0.00075 4.45524293434009e-09 397604.874033298 -614346.874646776;-0.000675 4.39152245928749e-09 414813.87544859 -602860.773675277;-0.0006 4.32429146837349e-09 431691.280998714 -590892.75502538;-0.000525 4.25360370502354e-09 448223.599143905 -578452.385748079;-0.00045 4.17951567595412e-09 464397.614201993 -565549.610484229;-0.000375 4.10208660600207e-09 480200.396912808 -552194.743514957;-0.0003 4.02137839078122e-09 495619.314773644 -538398.460516582;-0.000225 3.93745554720392e-09 510642.04213748 -524171.790026643;-0.00015 3.85038516190729e-09 525256.570065916 -509526.104627854;-7.5e-05 3.76023683762509e-09 539451.215928937 -494473.111857036]  x2=[-0.001275 1.59845903643484e-08 0 0;-0.0012 1.60013481609712e-08 0 0;-0.001125 1.6005314724703e-08 0 0;-0.00105 1.59964868847334e-08 0 0;-0.000975 1.59748716979025e-08 0 0;-0.0009 1.59404864430601e-08 0 0;-0.000825 1.58933586072527e-08 256317.712946236 -689303.964750558;-0.00075 1.58335258637513e-08 275702.267037893 -681782.177055932;-0.000675 1.57610360419354e-08 294866.428955666 -673715.383120584;-0.0006 1.56759470890595e-08 313794.87916174 -665110.031416161;-0.000525 1.55783270239307e-08 332472.486542634 -655973.000929149;-0.00045 1.54682538825354e-08 350884.320504786 -646311.595661917;-0.000375 1.53458156556585e-08 369015.662909836 -636133.538794013;-0.0003 1.52111102185454e-08 386852.019840086 -625446.966508366;-0.000225 1.50642452526614e-08 404379.133184709 -614260.421487351;-0.00015 1.49053381596131e-08 421582.992037473 -602582.8460839;-7.5e-05 1.47345159672993e-08 438449.843896838 -590423.575173115]  x3=[-0.001275 2.49144682867226e-11 0 0;-0.0012 2.76085770221595e-11 0 0;-0.001125 3.02806158835502e-11 0 0;-0.00105 3.29284488839125e-11 0 0;-0.000975 3.55499593860593e-11 0 0;-0.0009 3.81430517946054e-11 0 0;-0.000825 4.07056532311552e-11 504.220647790006 -2691.25110184037;-0.00075 4.32357151913293e-11 580.102277877287 -2675.92034911084;-0.000675 4.57312151823082e-11 655.520183079495 -2658.45050659718;-0.0006 4.81901583395813e-11 730.414075477145 -2638.8555394242;-0.000525 5.0610579021612e-11 804.724086038569 -2617.15111150885;-0.00045 5.29905423811406e-11 878.390812478305 -2593.35457303871;-0.000375 5.53281459118722e-11 951.355366742375 -2567.48494660255;-0.0003 5.76215209693109e-11 1023.5594220825 -2539.5629119839;-0.000225 5.98688342645255e-11 1094.94525968159 -2509.61078963003;-0.00015 6.2068289329653e-11 1165.45581479332 -2477.65252280927;-7.5e-05 6.4218127953967e-11 1235.03472235877 -2443.71365847112]  x4=[-0.001275 5.58738112353733e-11 0 0;-0.0012 5.36096306765177e-11 0 0;-0.001125 5.13025953991542e-11 0 0;-0.00105 4.89545496119846e-11 0 0;-0.000975 4.65673703068849e-11 0 0;-0.0009 4.41429657584666e-11 0 0;-0.000825 4.16832739986309e-11 4425.69676226999 -12765.9262438974;-0.00075 3.91902612673363e-11 4784.82745779851 -12635.706627188;-0.000675 3.66659204408156e-11 5140.13323546758 -12495.3862199337;-0.0006 3.41122694385019e-11 5491.33006927489 -12345.0771921209;-0.000525 3.15313496099344e-11 5838.13721784499 -12184.8996984868;-0.00045 2.89252241029344e-11 6180.27744884964 -12014.9817824689;-0.000375 2.62959762143574e-11 6517.4772606231 -11835.4592738495;-0.0003 2.36457077247365e-11 6849.46710079516 -11646.4756801752;-0.000225 2.09765372181519e-11 7175.98158176721 -11448.1820720392;-0.00015 1.8290598388667e-11 7496.75969285899 -11240.7369623178;-7.5e-05 1.55900383346856e-11 7811.54500895657 -11024.3061794579]  x5=0.00123288061605072  V1=ones(3,3)  V2=ones(3,3)  I1=ones(3,3)  I2=ones(3,3)  nHarmo=1  Measurements=None  Decoupling=on  VsMag0=[597501.495499285 597500.918482545 597501.873521954]  VrMag0=[600465.939453793 600465.308790945 600466.091594274]  VsAngle0=[19.1109154470688 -100.889010750014 139.11100026692]  VrAngle0=[8.21765611493073 -111.78229237891 128.21773398291]  IsMag0=[2247.1252586883 2247.11361991063 2247.12200887671]  IrMag0=[11088.6272022722 11088.6249727992 11088.6349972348]  IsAngle0=[-1.56829194736796 -121.568216294782 118.432002879331]  IrAngle0=[6.9404244715767 -113.059522369357 126.940461027589]
      settings: AttributesFormatString=\n  LibrarySourceBlock=sps_lib/Power Grid Elements/Distributed Parameters Line
  LMO7 : spsThreePhaseVIMeasurementLib/Three-Phase V-I Measurement  VoltageMeasurement=no  SetLabelV=on  LabelV=Vabc_LMO7  Vpu=on  VpuLL=off  CurrentMeasurement=no  SetLabelI=off  LabelI=A1  Ipu=off  Pbase=100e6  Vbase=735e3  OutputType=Magnitude  PhasorSimulation=off  PSBequivalent=0
  LVD 990 Mvar : spsThreePhaseSeriesRLCLoadLib/Three-Phase Series RLC Load  LConnTagsString=A|B|C  Configuration=Y (grounded)  NominalVoltage=735e3  Vabc=[1e3 1e3 1e3]  Vabcp=[1e3 1e3 1e3]  NominalFrequency=60  UnbalancedPower=off  ActivePower=3300000  InductivePower=990e6  CapacitivePower=0  Pabc=[10e3 9e3 11e3]  QLabc=[100 90 110]  QCabc=[100 90 110]  Pabcp=[10e3 9e3 11e3]  QLabcp=[100 90 110]  QCabcp=[100 90 110]  Measurements=None  LoadType=constant Z
  LVD-MTL 3*260km : spsDistributedParametersLineLib/Distributed Parameters Line  Phases=3  Length=260  Frequency=60  Resistance="[0.01273  0.3864]/3"  Inductance="[0.9337e-3  4.1264e-3]/3"  Capacitance=[12.74e-9 7.751e-9]*3  x1=[-0.0015 5.55590847231414e-08 -89258.2599346102 -744297.731345446;-0.001425 5.57521323348695e-08 -68180.8722481447 -746523.60785991;-0.00135 5.59006125450453e-08 -47048.9818156064 -748152.724824445;-0.001275 5.60044066608607e-08 -25879.4811468784 -749183.779947875;-0.0012 5.60634317108875e-08 -4689.29281689075 -749615.949020512;-0.001125 5.60776405114039e-08 16504.6440620261 -749448.88657301;-0.00105 5.60470217041122e-08 37685.3873810093 -748682.726152534;-0.000975 5.59715997652184e-08 58836.0055779258 -747318.080216001;-0.0009 5.58514349858665e-08 79939.5911722044 -745356.039640495;-0.000825 5.56866234239425e-08 100979.274280417 -742798.172851229;-0.00075 5.54772968272872e-08 121938.236101804 -739646.524567779;-0.000675 5.52236225283794e-08 142799.722362969 -735903.614169561;-0.0006 5.49258033105721e-08 163547.056710986 -731572.433681878;-0.000525 5.45840772459914e-08 184163.654044222 -726656.445384145;-0.00045 5.41987175052245e-08 204633.033770214 -721159.579042187;-0.000375 5.37700321389522e-08 224938.83298 -715086.228766855;-0.0003 5.32983638316971e-08 245064.819528382 -708441.249501432;-0.000225 5.27840896278873e-08 264994.90500965 -701229.953140673;-0.00015 5.22276206304525e-08 284713.157618411 -693458.104284551;-7.5e-05 5.16294016721952e-08 304203.81488523 -685131.915630129]  x2=[-0.0015 8.53736073503296e-08 -318141.458271989 -654659.491566498;-0.001425 8.55563571874613e-08 -299506.698691679 -663391.865921154;-0.00135 8.56707145817134e-08 -280632.51803904 -671593.934968429;-0.001275 8.57165881175348e-08 -261534.004045303 -679259.142099822;-0.0012 8.56939411243229e-08 -242226.423770337 -686381.359866033;-0.001125 8.56027917057374e-08 -222725.211398397 -692954.894875155;-0.00105 8.5443212725229e-08 -203045.955900275 -698974.492343879;-0.000975 8.52153317477931e-08 -183204.388571714 -704435.340298091;-0.0009 8.49193309379963e-08 -163216.370458049 -709333.073419492;-0.000825 8.45554469143569e-08 -143097.879675135 -713663.77653516;-0.00075 8.41239705601959e-08 -122864.99863668 -717423.987747289;-0.000675 8.36252467911091e-08 -102533.901198211 -720610.701200567;-0.0006 8.30596742792466e-08 -82120.8397279466 -723221.369485019;-0.000525 8.24277051346209e-08 -61642.1321148943 -725253.905672363;-0.00045 8.17298445436968e-08 -41114.1487245856 -726706.684984269;-0.000375 8.0966650365553e-08 -20553.2993128541 -727578.546091184;-0.0003 8.01387326859382e-08 23.9800918721885 -727868.792040679;-0.000225 7.92467533295781e-08 20601.2403272799 -727577.190814582;-0.00015 7.82914253311222e-08 41162.0322463795 -726703.975514453;-7.5e-05 7.72735123651557e-08 61689.9198667016 -725249.844175241]  x3=[-0.0015 2.44979879268808e-10 326.034617914316 -307.945403571588;-0.001425 2.53117305571415e-10 334.61041759937 -298.604572745246;-0.00135 2.61052393772774e-10 342.918734836307 -289.025041992254;-0.001275 2.68778800684786e-10 350.952928083448 -279.214469042926;-0.0012 2.76290349935984e-10 358.706574929639 -269.180696319169;-0.001125 2.83581036908828e-10 366.173477228226 -258.931744665377;-0.00105 2.90645033539702e-10 373.347666051759 -248.475806936689;-0.000975 2.97476692977782e-10 380.223406463461 -237.821241449742;-0.0009 3.04070554099042e-10 386.795202101649 -226.976565301168;-0.000825 3.10421345871791e-10 393.057799573442 -215.95044755915;-0.00075 3.16523991570256e-10 399.006192654242 -204.751702333505;-0.000675 3.22373612832839e-10 404.635626289634 -193.389281729822;-0.0006 3.27965533561805e-10 409.941600396502 -181.872268693279;-0.000525 3.33295283661283e-10 414.919873460331 -170.209869747881;-0.00045 3.3835860261059e-10 419.566465925802 -158.411407636905;-0.000375 3.43151442870031e-10 423.877663377994 -146.48631387044;-0.0003 3.47669973116435e-10 427.850019511628 -134.444121185983;-0.000225 3.51910581305859e-10 431.480358885989 -122.294455928114;-0.00015 3.55869877560999e-10 434.765779463327 -110.047030353344;-7.5e-05 3.59544696881009e-10 437.703654928702 -97.7116348662855]  x4=[-0.0015 2.60498644847016e-10 -7428.61939570774 -14286.1681180438;-0.001425 2.57972354833421e-10 -7021.77252832251 -14490.4696992911;-0.00135 2.55239845666483e-10 -6609.31256341487 -14683.1878207725;-0.001275 2.52303301672219e-10 -6191.5692151699 -14864.1684265702;-0.0012 2.49165070278968e-10 -5768.87642122851 -15033.2668435571;-0.001125 2.4582766014089e-10 -5341.57207574276 -15190.3478970459;-0.00105 2.42293739132584e-10 -4909.99775926845 -15335.286018846;-0.000975 2.38566132216434e-10 -4474.49846571087 -15467.9653476404;-0.0009 2.34647819184375e-10 -4035.42232654193 -15588.2798216037;-0.000825 2.30541932275892e-10 -3593.12033250917 -15696.1332631862;-0.00075 2.26251753674157e-10 -3147.9460530592 -15791.4394559971;-0.000675 2.21780712882303e-10 -2700.2553536996 -15874.1222137239;-0.0006 2.1713238398193e-10 -2250.40611152554 -15944.1154410353;-0.000525 2.12310482776038e-10 -1798.7579291383 -16001.3631864163;-0.00045 2.07318863818674e-10 -1345.67184718442 -16045.8196868952;-0.000375 2.02161517333659e-10 -891.510055745378 -16077.4494046256;-0.0003 1.96842566024863e-10 -436.635604808331 -16096.2270552952;-0.000225 1.91366261780578e-10 18.5878859504508 -16102.1376283373;-0.00015 1.85736982274628e-10 473.796517837608 -16095.1763989303;-7.5e-05 1.79959227466918e-10 928.626404037736 -16075.3489317745]  x5=0.00147040807418893  V1=ones(3,3)  V2=ones(3,3)  I1=ones(3,3)  I2=ones(3,3)  nHarmo=1  Measurements=None  Decoupling=on  VsMag0=[612070.91918421 612070.526870902 612070.832121352]  VrMag0=[594302.518281082 594302.525591459 594302.380387509]  VsAngle0=[-4.43840982432267 -124.438398032262 115.561627875916]  VrAngle0=[-23.5181046800034 -143.518120437634 96.481886830827]  IsMag0=[368.438417398339 368.42277858594 368.434712935229]  IrMag0=[13227.9520808209 13227.9561692171 13227.964922959]  IsAngle0=[49.0336389582177 -70.9656221604626 169.036114575817]  IrAngle0=[-25.07389132503 -145.073837319249 94.9261203418274]
      settings: AttributesFormatString=\n  LibrarySourceBlock=sps_lib/Power Grid Elements/Distributed Parameters Line
  LVD7 : spsThreePhaseVIMeasurementLib/Three-Phase V-I Measurement  VoltageMeasurement=no  SetLabelV=on  LabelV=Vabc_LVD7  Vpu=on  VpuLL=off  CurrentMeasurement=no  SetLabelI=off  LabelI=A1  Ipu=off  Pbase=100e6  Vbase=735e3  OutputType=Magnitude  PhasorSimulation=off  PSBequivalent=0
  Load Flow Bus1 : spsLoadFlowBusLib/Load Flow Bus  LConnTagsString=a  Phases=single  Connectors=on one side  ID=LG31_13.8  Vbase=13.8e3  Vref=1  Vangle=0  VLF=1  VLFb=1  VLFc=1  angleLF=-0.0351  angleLFb=0  angleLFc=0
      settings: AttributesFormatString=%<ID>\n%<Vbase>V\n%<VLF>pu\n%<angleLF>deg.
  Load Flow Bus10 : spsLoadFlowBusLib/Load Flow Bus  LConnTagsString=a  Phases=single  Connectors=on one side  ID=LVD7  Vbase=735e3  Vref=1  Vangle=0  VLF=1.05  VLFb=1  VLFc=1  angleLF=-12.02  angleLFb=0  angleLFc=0
      settings: AttributesFormatString=%<ID>\n%<Vbase>V\n%<VLF>pu\n%<angleLF>deg.
  Load Flow Bus11 : spsLoadFlowBusLib/Load Flow Bus  LConnTagsString=a  Phases=single  Connectors=on one side  ID=CHM7  Vbase=735e3  Vref=1  Vangle=0  VLF=1.047  VLFb=1  VLFc=1  angleLF=-4.064  angleLFb=0  angleLFc=0
      settings: AttributesFormatString=%<ID>\n%<Vbase>V\n%<VLF>pu\n%<angleLF>deg.
  Load Flow Bus12 : spsLoadFlowBusLib/Load Flow Bus  LConnTagsString=a  Phases=single  Connectors=on one side  ID=LG47  Vbase=735e3  Vref=1  Vangle=0  VLF=1.004  VLFb=1  VLFc=1  angleLF=20.71  angleLFb=0  angleLFc=0
      settings: AttributesFormatString=%<ID>\n%<Vbase>V\n%<VLF>pu\n%<angleLF>deg.
  Load Flow Bus2 : spsLoadFlowBusLib/Load Flow Bus  LConnTagsString=a  Phases=single  Connectors=on one side  ID=LG3_13.8  Vbase=13.8e3  Vref=1  Vangle=0  VLF=1  VLFb=1  VLFc=1  angleLF=-0.6025  angleLFb=0  angleLFc=0
      settings: AttributesFormatString=%<ID>\n%<Vbase>V\n%<VLF>pu\n%<angleLF>deg.
  Load Flow Bus3 : spsLoadFlowBusLib/Load Flow Bus  LConnTagsString=a  Phases=single  Connectors=on one side  ID=LG4_13.8  Vbase=13.8e3  Vref=1  Vangle=0  VLF=1  VLFb=1  VLFc=1  angleLF=-3.293  angleLFb=0  angleLFc=0
      settings: AttributesFormatString=%<ID>\n%<Vbase>V\n%<VLF>pu\n%<angleLF>deg.
  Load Flow Bus4 : spsLoadFlowBusLib/Load Flow Bus  LConnTagsString=a  Phases=single  Connectors=on one side  ID=LG2_13.8  Vbase=13.8e3  Vref=1  Vangle=0  VLF=1  VLFb=1  VLFc=1  angleLF=0  angleLFb=0  angleLFc=0
      settings: AttributesFormatString=%<ID>\n%<Vbase>V\n%<VLF>pu\n%<angleLF>deg.
  Load Flow Bus5 : spsLoadFlowBusLib/Load Flow Bus  LConnTagsString=a  Phases=single  Connectors=on one side  ID=LG27  Vbase=735e3  Vref=1  Vangle=0  VLF=1  VLFb=1  VLFc=1  angleLF=23.57  angleLFb=0  angleLFc=0
      settings: AttributesFormatString=%<ID>\n%<Vbase>V\n%<VLF>pu\n%<angleLF>deg.
  Load Flow Bus6 : spsLoadFlowBusLib/Load Flow Bus  LConnTagsString=a  Phases=single  Connectors=on one side  ID=LG37  Vbase=735e3  Vref=1  Vangle=0  VLF=0.994  VLFb=1  VLFc=1  angleLF=24.1  angleLFb=0  angleLFc=0
      settings: AttributesFormatString=%<ID>\n%<Vbase>V\n%<VLF>pu\n%<angleLF>deg.
  Load Flow Bus7 : spsLoadFlowBusLib/Load Flow Bus  LConnTagsString=a  Phases=single  Connectors=on one side  ID=LMO7  Vbase=735e3  Vref=1  Vangle=0  VLF=1.016  VLFb=1  VLFc=1  angleLF=17.31  angleLFb=0  angleLFc=0
      settings: AttributesFormatString=%<ID>\n%<Vbase>V\n%<VLF>pu\n%<angleLF>deg.
  Load Flow Bus8 : spsLoadFlowBusLib/Load Flow Bus  LConnTagsString=a  Phases=single  Connectors=on one side  ID=NEM_ALB7  Vbase=735e3  Vref=1  Vangle=0  VLF=1.028  VLFb=1  VLFc=1  angleLF=8.928  angleLFb=0  angleLFc=0
      settings: AttributesFormatString=%<ID>\n%<Vbase>V\n%<VLF>pu\n%<angleLF>deg.
  Load Flow Bus9 : spsLoadFlowBusLib/Load Flow Bus  LConnTagsString=a  Phases=single  Connectors=on one side  ID=ABI_CHB7  Vbase=735e3  Vref=1  Vangle=0  VLF=1.046  VLFb=1  VLFc=1  angleLF=0.1334  angleLFb=0  angleLFc=0
      settings: AttributesFormatString=%<ID>\n%<Vbase>V\n%<VLF>pu\n%<angleLF>deg.
  NEM-ABI 6*236 : spsDistributedParametersLineLib/Distributed Parameters Line  Phases=3  Length=236  Frequency=60  Resistance="[0.01273  0.3864]/6"  Inductance="[0.9337e-3  4.1264e-3]/6"  Capacitance=[12.74e-9 7.751e-9]*6  x1=[-0.00135 1.5518946135204e-08 0 0;-0.001275 1.55606207636779e-08 0 0;-0.0012 1.55898564699988e-08 0 0;-0.001125 1.56066298835904e-08 0 0;-0.00105 1.56109275960425e-08 0 0;-0.000975 1.56027461718296e-08 0 0;-0.0009 1.55820921510568e-08 0 0;-0.000825 1.55489820442326e-08 284117.477880577 -680689.106292241;-0.00075 1.55034423190695e-08 303247.373018719 -672384.845537271;-0.000675 1.54455093793273e-08 322134.856846709 -663543.090624613;-0.0006 1.53752295357114e-08 340764.830998965 -654170.909517859;-0.000525 1.52926589688536e-08 359122.402959197 -644275.794195187;-0.00045 1.51978636844016e-08 377192.897965261 -633865.654660385;-0.000375 1.50909194602554e-08 394961.870739936 -622948.812619718;-0.0003 1.49719117859914e-08 412415.117038261 -611533.994829679;-0.000225 1.48409357945237e-08 429538.685002188 -599630.326120957;-0.00015 1.46980961860558e-08 446318.886313486 -587247.322104185;-7.5e-05 1.45435071443852e-08 462742.307135974 -574394.881563309]  x2=[-0.00135 2.79928488076701e-08 0 0;-0.001275 2.80425733483352e-08 0 0;-0.0012 2.80698810849315e-08 0 0;-0.001125 2.8074750188072e-08 0 0;-0.00105 2.80571767654703e-08 0 0;-0.000975 2.80171748650515e-08 0 0;-0.0009 2.79547764637227e-08 0 0;-0.000825 2.78700314418112e-08 125357.104454003 -735061.346285092;-0.00075 2.77630075431909e-08 146087.597415348 -731223.617197145;-0.000675 2.76337903211289e-08 166701.310186535 -726801.359137708;-0.0006 2.74824830698953e-08 187181.764480974 -721798.107192209;-0.000525 2.73092067421917e-08 207512.588536864 -716217.860883703;-0.00045 2.71140998524633e-08 227677.530204526 -710065.080975707;-0.000375 2.68973183661725e-08 247660.469938127 -703344.685906339;-0.0003 2.66590355751225e-08 267445.43368139 -696062.047856592;-0.000225 2.63994419589307e-08 287016.605637022 -688222.988455895;-0.00015 2.61187450327619e-08 306358.340909608 -679833.774128391;-7.5e-05 2.58171691814442e-08 325455.178011912 -670901.111083654]  x3=[-0.00135 1.52640233576614e-10 0 0;-0.001275 1.59122042707421e-10 0 0;-0.0012 1.65476652111936e-10 0 0;-0.001125 1.7169898201263e-10 0 0;-0.00105 1.77784058374186e-10 0 0;-0.000975 1.83727016879665e-10 0 0;-0.0009 1.89523106818968e-10 0 0;-0.000825 1.9516769488648e-10 -448.187482109962 -4499.57322110024;-0.00075 2.00656268884866e-10 -320.801895602993 -4510.44404860237;-0.000675 2.0598444133205e-10 -193.159864969113 -4517.70929614416;-0.0006 2.111479529685e-10 -65.3634252946209 -4521.36315599788;-0.000525 2.16142676162019e-10 62.4852649019573 -4521.40270732386;-0.00045 2.20964618207309e-10 190.28400533383 -4517.8279185054;-0.000375 2.25609924517675e-10 317.930635643281 -4510.64164717397;-0.0003 2.3007488170633e-10 445.323117067101 -4499.84963792492;-0.000225 2.34355920554812e-10 572.35961400481 -4485.46051772532;-0.00015 2.38449618866168e-10 698.938575424479 -4467.48578901769;-7.5e-05 2.42352704200605e-10 824.958816041073 -4445.93982052515]  x4=[-0.00135 1.61545911133686e-10 0 0;-0.001275 1.5805514831217e-10 0 0;-0.0012 1.54438038623418e-10 0 0;-0.001125 1.50697473529572e-10 0 0;-0.00105 1.46836443181135e-10 0 0;-0.000975 1.42858034026691e-10 0 0;-0.0009 1.38765426345648e-10 0 0;-0.000825 1.34561891705967e-10 4622.22438525129 -28011.6084746989;-0.00075 1.30250790348922e-10 5412.27949589202 -27869.7398149581;-0.000675 1.25835568502975e-10 6198.00811311439 -27705.5925116305;-0.0006 1.21319755628916e-10 6978.78213748384 -27519.2977815589;-0.000525 1.16706961598462e-10 7753.97743019153 -27311.0045459001;-0.00045 1.12000873808583e-10 8522.97431198136 -27080.8793110797;-0.000375 1.07205254233852e-10 9285.15805851207 -26829.1060356893;-0.0003 1.02323936419181e-10 10039.9193917585 -26555.8859834331;-0.000225 9.73608224153463e-11 10786.6549670591 -26261.4375622405;-0.00015 9.23198796597429e-11 11524.7678554203 -25945.996149674;-7.5e-05 8.72051378048811e-11 12253.6680206928 -25609.8139047726]  x5=0.00133467809810995  V1=ones(3,3)  V2=ones(3,3)  I1=ones(3,3)  I2=ones(3,3)  nHarmo=1  Measurements=None  Decoupling=on  VsMag0=[602251.717194415 602251.086049868 602251.913986952]  VrMag0=[608840.309919351 608839.972623173 608840.270927492]  VsAngle0=[10.47550453193 -109.524439182988 130.475584674523]  VrAngle0=[-2.50190241955592 -122.501888330505 117.498132114117]  IsMag0=[3712.64388956013 3712.615218024 3712.60597455712]  IrMag0=[23309.611878834 23309.6245706263 23309.6488489252]  IsAngle0=[-17.8678983044547 -137.86831849006 102.132274803431]  IrAngle0=[-2.81003503241819 -122.809948112046 117.189981410571]
      settings: AttributesFormatString=\n  LibrarySourceBlock=sps_lib/Power Grid Elements/Distributed Parameters Line
  NEM-ALB 1980 Mvar : spsThreePhaseSeriesRLCLoadLib/Three-Phase Series RLC Load  LConnTagsString=A|B|C  Configuration=Y (grounded)  NominalVoltage=735e3  Vabc=[1e3 1e3 1e3]  Vabcp=[1e3 1e3 1e3]  NominalFrequency=60  UnbalancedPower=off  ActivePower=6600000  InductivePower=1980e6  CapacitivePower=0  Pabc=[10e3 9e3 11e3]  QLabc=[100 90 110]  QCabc=[100 90 110]  Pabcp=[10e3 9e3 11e3]  QLabcp=[100 90 110]  QCabcp=[100 90 110]  Measurements=None  LoadType=constant Z
  NEM-ALB7 : spsThreePhaseVIMeasurementLib/Three-Phase V-I Measurement  VoltageMeasurement=no  SetLabelV=on  LabelV=Vabc_NEM7  Vpu=on  VpuLL=off  CurrentMeasurement=no  SetLabelI=off  LabelI=A1  Ipu=off  Pbase=100e6  Vbase=735e3  OutputType=Magnitude  PhasorSimulation=off  PSBequivalent=0
  Regulators1 : Subsystem
  Regulators2 : Subsystem
  Regulators3 : Subsystem
  Regulators4 : Subsystem
  MTLa : PMIOPort  Side=Right
  MTLb : PMIOPort  Port=2  Side=Right
  MTLc : PMIOPort  Port=3  Side=Right
  CHM7a : PMIOPort  Port=4  Side=Right
  CHM7b : PMIOPort  Port=5  Side=Right
  CHM7c : PMIOPort  Port=6  Side=Right
  wires:
  Regulators2/1(Pm) -> LG3_2200 MVA/1
  Regulators4/2(Vf) -> LG4-2700 MVA/2
  Regulators4/1(Pm) -> LG4-2700 MVA/1
  Regulators3/2(Vf) -> LG31-200 MVA/2
  Regulators3/1(Pm) -> LG31-200 MVA/1
  Regulators2/2(Vf) -> LG3_2200 MVA/2
  LG3_2200 MVA/1 -> Regulators2/1(m)
  Regulators1/1(Pm) -> LG2_5500 MVA/1
  Regulators1/2(Vf) -> LG2_5500 MVA/2
  LG2_5500 MVA/1 -> Regulators1/1(m)
  LG31-200 MVA/1 -> Regulators3/1(m)
  LG4-2700 MVA/1 -> Regulators4/1(m)
  connections:
  LG2-NENI 3*279km/RConn1 -- "Cs NEM "/LConn1
  LG2-NENI 3*279km/RConn2 -- "Cs NEM "/LConn2
  LG2-NENI 3*279km/RConn3 -- "Cs NEM "/LConn3
  CHB-CHM 3*195km/RConn1 -- "Cs  CHMN "/LConn1
  CHB-CHM 3*195km/RConn2 -- "Cs  CHMN "/LConn2
  CHB-CHM 3*195km/RConn3 -- "Cs  CHMN "/LConn3
  Load Flow Bus2/LConn1 -- 2200 MVA 13.8 kV/735 kV/LConn1 -- LG3_2200 MVA/RConn1 -- 110 MW/LConn1
  2200 MVA 13.8 kV/735 kV/LConn2 -- LG3_2200 MVA/RConn2 -- 110 MW/LConn2
  2200 MVA 13.8 kV/735 kV/LConn3 -- LG3_2200 MVA/RConn3 -- 110 MW/LConn3
  Load Flow Bus1/LConn1 -- 200 MVA 13.8 kV/735 kV/LConn1 -- LG31-200 MVA/RConn1 -- 10 MW/LConn1
  200 MVA 13.8 kV/735 kV/LConn2 -- LG31-200 MVA/RConn2 -- 10 MW/LConn2
  200 MVA 13.8 kV/735 kV/LConn3 -- LG31-200 MVA/RConn3 -- 10 MW/LConn3
  Load Flow Bus6/LConn1 -- 2200 MVA 13.8 kV/735 kV/RConn1 -- 200 MVA 13.8 kV/735 kV/RConn1 -- LG3-LMO 104km/LConn1 -- LG3 660 Mvar/LConn1 -- LG2-LG3 155km/RConn1
  2200 MVA 13.8 kV/735 kV/RConn2 -- LG3 660 Mvar/LConn2 -- LG2-LG3 155km/RConn2 -- 200 MVA 13.8 kV/735 kV/RConn2 -- LG3-LMO 104km/LConn2
  LG3-LMO 104km/RConn1 -- LMO7/RConn1 -- LG4-LMO 3*118km/RConn1 -- LMO 330 Mvar/LConn1
  LG3-LMO 104km/RConn2 -- LMO7/RConn2 -- LG4-LMO 3*118km/RConn2 -- LMO 330 Mvar/LConn2
  LG3-LMO 104km/RConn3 -- LMO7/RConn3 -- LG4-LMO 3*118km/RConn3 -- LMO 330 Mvar/LConn3
  LG4-LMO 3*118km/LConn1 -- LG4 660 Mvar/LConn1 -- 2700 MVA 13.8 kV/735 kV/RConn1 -- Load Flow Bus12/LConn1
  LG4-LMO 3*118km/LConn2 -- 2700 MVA 13.8 kV/735 kV/RConn2 -- LG4 660 Mvar/LConn2
  LG4 660 Mvar/LConn3 -- 2700 MVA 13.8 kV/735 kV/RConn3 -- LG4-LMO 3*118km/LConn3
  Load Flow Bus3/LConn1 -- LG4-2700 MVA/RConn1 -- 2700 MVA 13.8 kV/735 kV/LConn1 -- 135 MW/LConn1
  LG4-2700 MVA/RConn2 -- 2700 MVA 13.8 kV/735 kV/LConn2 -- 135 MW/LConn2
  LG4-2700 MVA/RConn3 -- 2700 MVA 13.8 kV/735 kV/LConn3 -- 135 MW/LConn3
  Load Flow Bus4/LConn1 -- 5500 MVA 13.8 kV/735 kV/LConn1 -- LG2_5500 MVA/RConn1 -- 275 MW/LConn1
  5500 MVA 13.8 kV/735 kV/LConn2 -- LG2_5500 MVA/RConn2 -- 275 MW/LConn2
  LG2_5500 MVA/RConn3 -- 5500 MVA 13.8 kV/735 kV/LConn3 -- 275 MW/LConn3
  5500 MVA 13.8 kV/735 kV/RConn1 -- LG2-NENI 3*279km/LConn1 -- LG2-LG3 155km/LConn1 -- LG2 660 Mvar/LConn1 -- Load Flow Bus5/LConn1
  LG2-LG3 155km/LConn2 -- 5500 MVA 13.8 kV/735 kV/RConn2 -- LG2-NENI 3*279km/LConn2 -- LG2 660 Mvar/LConn2
  LG2-LG3 155km/LConn3 -- 5500 MVA 13.8 kV/735 kV/RConn3 -- LG2-NENI 3*279km/LConn3 -- LG2 660 Mvar/LConn3
  "Cs NEM "/RConn1 -- NEM-ALB7/LConn1 -- Cs ALB/RConn1
  "Cs NEM "/RConn2 -- NEM-ALB7/LConn2 -- Cs ALB/RConn2
  "Cs NEM "/RConn3 -- NEM-ALB7/LConn3 -- Cs ALB/RConn3
  LMO7/LConn1 -- LMO-ALB 3*218km/LConn1
  LMO7/LConn2 -- LMO-ALB 3*218km/LConn2
  Load Flow Bus7/LConn1 -- LMO7/LConn3 -- LMO-ALB 3*218km/LConn3
  Cs ALB/LConn1 -- LMO-ALB 3*218km/RConn1
  Cs ALB/LConn2 -- LMO-ALB 3*218km/RConn2
  Cs ALB/LConn3 -- LMO-ALB 3*218km/RConn3
  200 MVA 13.8 kV/735 kV/RConn3 -- LG3-LMO 104km/LConn3 -- LG3 660 Mvar/LConn3 -- LG2-LG3 155km/RConn3 -- 2200 MVA 13.8 kV/735 kV/RConn3
  Load Flow Bus8/LConn1 -- NEM-ABI 6*236/LConn1 -- NEM-ALB7/RConn1 -- NEM-ALB 1980 Mvar/LConn1
  NEM-ALB 1980 Mvar/LConn2 -- NEM-ALB7/RConn2 -- NEM-ABI 6*236/LConn2
  NEM-ALB 1980 Mvar/LConn3 -- NEM-ALB7/RConn3 -- NEM-ABI 6*236/LConn3
  NEM-ABI 6*236/RConn1 -- "Cs ABI+CHB "/LConn1
  NEM-ABI 6*236/RConn2 -- "Cs ABI+CHB "/LConn2
  NEM-ABI 6*236/RConn3 -- "Cs ABI+CHB "/LConn3
  "Cs ABI+CHB "/RConn1 -- ABI-CHB7/LConn1
  "Cs ABI+CHB "/RConn2 -- ABI-CHB7/LConn2
  "Cs ABI+CHB "/RConn3 -- ABI-CHB7/LConn3
  Load Flow Bus9/LConn1 -- ABI+CHB 1320 Mvar/LConn1 -- CHB-CHM 3*195km/LConn1 -- ABI-CHB 3*271km/LConn1 -- ABI-CHB7/RConn1
  ABI-CHB 3*271km/LConn2 -- ABI-CHB7/RConn2 -- ABI+CHB 1320 Mvar/LConn2 -- CHB-CHM 3*195km/LConn2
  ABI-CHB 3*271km/LConn3 -- ABI-CHB7/RConn3 -- ABI+CHB 1320 Mvar/LConn3 -- CHB-CHM 3*195km/LConn3
  ABI-CHB 3*271km/RConn1 -- "Cs LVDN "/LConn1
  ABI-CHB 3*271km/RConn2 -- "Cs LVDN "/LConn2
  ABI-CHB 3*271km/RConn3 -- "Cs LVDN "/LConn3
  "Cs LVDN "/RConn1 -- LVD7/LConn1
  "Cs LVDN "/RConn2 -- LVD7/LConn2
  "Cs LVDN "/RConn3 -- LVD7/LConn3
  "Cs LVDS "/LConn1 -- LVD 990 Mvar/LConn1 -- Load Flow Bus10/LConn1 -- LVD7/RConn1
  "Cs LVDS "/LConn2 -- LVD7/RConn2 -- LVD 990 Mvar/LConn2
  "Cs LVDS "/LConn3 -- LVD7/RConn3 -- LVD 990 Mvar/LConn3
  "Cs LVDS "/RConn1 -- LVD-MTL 3*260km/LConn1
  "Cs LVDS "/RConn2 -- LVD-MTL 3*260km/LConn2
  "Cs LVDS "/RConn3 -- LVD-MTL 3*260km/LConn3
  MTLa/RConn1 -- LVD-MTL 3*260km/RConn1
  MTLb/RConn1 -- LVD-MTL 3*260km/RConn2
  MTLc/RConn1 -- LVD-MTL 3*260km/RConn3
  "Cs  CHMN "/RConn1 -- CHM7/LConn1
  "Cs  CHMN "/RConn2 -- CHM7/LConn2
  "Cs  CHMN "/RConn3 -- CHM7/LConn3
  CHM 1320Mvar/LConn2 -- CHM7/RConn2 -- CHM7b/RConn1
  Load Flow Bus11/LConn1 -- CHM 1320Mvar/LConn3 -- CHM7c/RConn1 -- CHM7/RConn3
  CHM7a/RConn1 -- CHM 1320Mvar/LConn1 -- CHM7/RConn1
